simulink model "state_space_simulink_compare"  (R2016b)
settings: Solver=VariableStepAuto  StartTime=0.0  StopTime=2.0  RelTol=1e-3
values from neighbouring files (symbols this model uses):
  A = [ 0   1   0 ... (first row only)    [test_stateSpace.m]
  B = [ 0 ... (first row only)    [test_stateSpace.m]
  C = [ 1 0 0; eye(3)]    [test_stateSpace.m]
  D = zeros ( size (C, 1), size (B, 2) )    [test_stateSpace.m]
  K = [-280.7143e+000 , -7.7857e+000,  -300.0000e-003]    [test_stateSpace.m]
  x0 = [0.01 0 0]    [test_stateSpace.m]
settings Model: Creator=rcrozier  LastModifiedBy=rcrozier

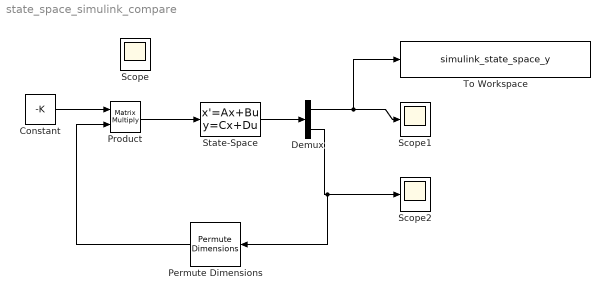
== system state_space_simulink_compare ==
  Constant : Constant  Value=-K  VectorParams1D=off
  Demux : Demux  Outputs=[ 1, 3]
  Permute Dimensions : PermuteDimensions
  Product : Product  Multiplication=Matrix(*)
  Scope1 : Scope
  Scope2 : Scope
  State-Space : StateSpace  A=A  B=B  C=C  D=D  X0=x0  ContinuousStateAttributes='x'
  To Workspace : ToWorkspace  VariableName=simulink_state_space_y  SaveFormat=Structure With Time  SampleTime=-1
  Scope : Scope
  wires:
  Constant/1 -> Product/1
  State-Space/1 -> Demux/1
  Demux/2 -> Permute Dimensions/1, Scope2/1
  Product/1 -> State-Space/1
  Demux/1 -> To Workspace/1, Scope1/1
  Permute Dimensions/1 -> Product/2
